simulink model "realtime_pacer_example"  (Simulink 10.0)
settings: Solver=ode3  StartTime=0.0  StopTime=5  FixedStep=0.05  RelTol=1e-3  EnableMultiTasking=on
model workspace (MAT data in the model file):
  Var : num (value not decoded)
libraries: realtime_pacer_lib x2
settings Model: Creator=gvallabh  LastModifiedBy=bhisma
settings DataIOCC: LimitDataPoints=on  SignalLoggingSaveFormat=ModelDataLogs
settings OptimizationCC: ExpressionDepthLimit=2147483647
settings DebuggingCC: SolverPrmCheckMsg=warning  FcnCallInpInsideContextMsg=warning  StateNameClashWarn=warning
settings GRTTargetCC: GeneratePreprocessorConditionals=Disable all
settings ConfigComp: CovExternalEMLEnable=off

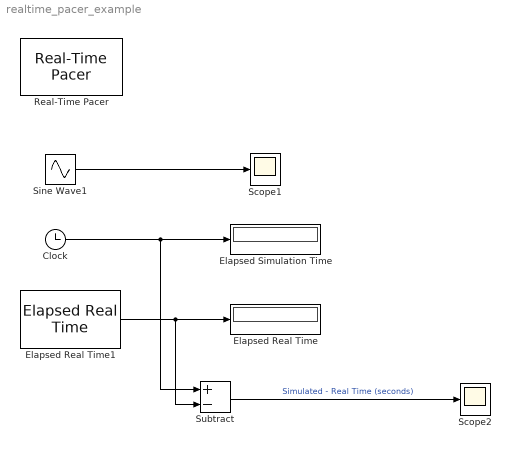
== system realtime_pacer_example ==
  Clock : Clock
  Elapsed Real Time : Display
      settings: Decimation=2
  Elapsed Real Time1 : realtime_pacer_lib/Elapsed Real Time
  Elapsed Simulation Time : Display
      settings: Decimation=2
  Real-Time Pacer : realtime_pacer_lib/Real-Time Pacer  simTimePerRealTime=1
  Scope1 : Scope
  Scope2 : Scope
  Sine Wave1 : Sin  Frequency=2*pi*0.5  SampleTime=0
  Subtract : Sum  Inputs=+-
  wires:
  Clock/1 -> Elapsed Simulation Time/1, Subtract/1
  Sine Wave1/1 -> Scope1/1
  Subtract/1 -> Scope2/1  "Simulated - Real Time (seconds)"
  Elapsed Real Time1/1 -> Elapsed Real Time/1, Subtract/2
